simulink model "T2_Full_sim"  (R2023b)
settings: Solver=FixedStepAuto  StartTime=0.0  StopTime=Tf  FixedStep=Ts/100  MaxStep=1e-5  RelTol=1e-3
undefined symbols (not defined in the file): A_KF, AA, AAlim, Ad_KF, BB, bblim, C, C_KF, C_KF_ROT, EE, KF, KF_ROT, L, lambda_u, Mx, N, nH, plecs, R, ref_ROT, Ts, Vdc, Vo, W, w, x_ROT
libraries: spsAlphaBetaZerotoabcLib x6
settings Model: Creator=lokit  LastModifiedBy=pablo

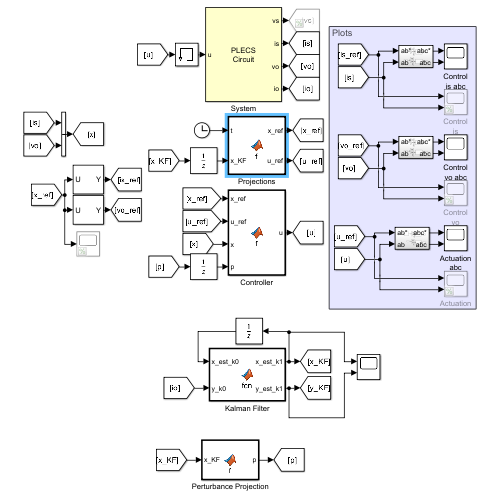
[thumbnail: Simulink's stored preview of the top-level diagram]
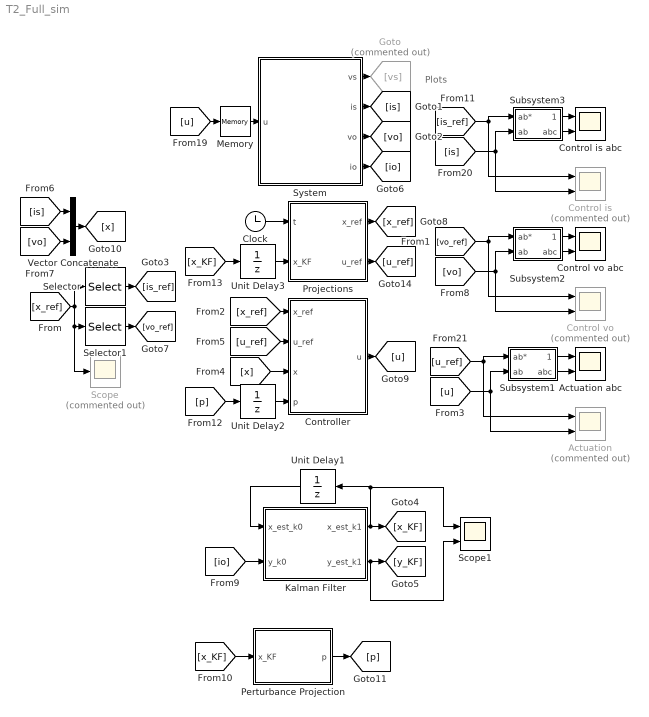
== system T2_Full_sim ==
  note: Plots
  Actuation : Scope  Commented=on  NumInputPorts=2
  Actuation abc : Scope  NumInputPorts=2
  Clock : Clock
  Control is : Scope  Commented=on  NumInputPorts=2
  Control is abc : Scope  NumInputPorts=2
  Control vo : Scope  Commented=on  NumInputPorts=2
  Control vo abc : Scope  NumInputPorts=2
  Controller : MATLAB Function  TreatAsAtomicUnit=on  SystemSampleTime=Ts
  Goto : Goto  Commented=on  GotoTag=vs
  Kalman Filter : MATLAB Function  TreatAsAtomicUnit=on  SystemSampleTime=Ts
  Memory : Memory
  Perturbance Projection : MATLAB Function  TreatAsAtomicUnit=on  SystemSampleTime=Ts
  Projections : MATLAB Function  TreatAsAtomicUnit=on  SystemSampleTime=Ts
  Scope : Scope  Commented=on
  Scope1 : Scope  NumInputPorts=2
  Selector : Selector  InputPortWidth=4*N  IndexOptions=Index vector (dialog)  Indices=[1 2]  OutputSizes=1
  Selector1 : Selector  InputPortWidth=4*N  IndexOptions=Index vector (dialog)  Indices=[3 4]  OutputSizes=1
  Subsystem1 : Subsystem
  Subsystem2 : Subsystem
  Subsystem3 : Subsystem
  System : Subsystem  LoadFcn=plecs('sl', 200);  InitFcn=plecs('sl', 214);  StartFcn=plecs('sl', 208);  StopFcn=plecs('sl', 209);  mask(PlecsCircuit){PLECSData=<binary blob, 8800 chars, not shown>}
      mask prompts: PLECSData "PLECS Data (Do not delete or modify!)"
      mask init:
      | % PLACE CUSTOM INITIALIZATIONS ABOVE
      | % DO NOT REMOVE
      | plecs('sl', 215);
      | % DO NOT REMOVE
      settings: CopyFcn=plecs('sl', 203);  DeleteFcn=plecs('sl', 205);  UndoDeleteFcn=plecs('sl', 206);  PreSaveFcn=plecs('sl', 211);  PostSaveFcn=plecs('sl', 201);  NameChangeFcn=plecs('sl', 210);  DestroyFcn=plecs('sl', 207);  PreCopyFcn=plecs('sl', 216);  OpenFcn=plecs('sl', 202);  ErrorFcn=plerrorfcn
      mask Help: eval('plecs(''help'', ''qthelp:///creatingacircuit.html'')')
      mask Display: disp('PLECS\nCircuit')
  Unit Delay1 : UnitDelay  InitialCondition=zeros(nH, 1)  SampleTime=Ts  HasFrameUpgradeWarning=on
  Unit Delay2 : UnitDelay  SampleTime=Ts  HasFrameUpgradeWarning=on
  Unit Delay3 : UnitDelay  SampleTime=Ts  HasFrameUpgradeWarning=on
  Vector Concatenate : Concatenate
  wires:
  Projections/1(x_ref) -> [x_ref]
  Clock/1 -> Projections/1(t)
  Controller/1(u) -> [u]
  [x_ref] -> Controller/1(x_ref)
  [x] -> Controller/3(x)
  [is] -> Vector Concatenate/1
  [vo] -> Vector Concatenate/2
  Vector Concatenate/1 -> [x]
  Projections/2(u_ref) -> [u_ref]
  [u_ref] -> Controller/2(u_ref)
  [u_ref] -> Subsystem1/1(ab*), Actuation/1
  Subsystem1/2(abc) -> Actuation abc/2
  Subsystem1/1(abc*) -> Actuation abc/1
  [u] -> Actuation/2, Subsystem1/2(ab)
  Selector/1 -> [is_ref]
  [x_ref] -> Scope/1, Selector1/1, Selector/1
  Subsystem2/2(abc) -> Control vo abc/2
  [vo_ref] -> Control vo/1, Subsystem2/1(ab*)
  [vo] -> Control vo/2, Subsystem2/2(ab)
  Subsystem2/1(abc*) -> Control vo abc/1
  Subsystem3/2(abc) -> Control is abc/2
  [is_ref] -> Control is/1, Subsystem3/1(ab*)
  [is] -> Subsystem3/2(ab), Control is/2
  Subsystem3/1(abc*) -> Control is abc/1
  Selector1/1 -> [vo_ref]
  System/4(io) -> [io]
  System/1(vs) -> Goto/1
  Memory/1 -> System/1(u)
  [u] -> Memory/1
  System/3(vo) -> [vo]
  System/2(is) -> [is]
  Kalman Filter/1(x_est_k1) -> Scope1/1, Unit Delay1/1, [x_KF]
  Kalman Filter/2(y_est_k1) -> Scope1/2, [y_KF]
  [io] -> Kalman Filter/2(y_k0)
  Unit Delay1/1 -> Kalman Filter/1(x_est_k0)
  [x_KF] -> Perturbance Projection/1(x_KF)
  [p] -> Unit Delay2/1
  Perturbance Projection/1(p) -> [p]
  [x_KF] -> Unit Delay3/1
  Unit Delay3/1 -> Projections/2(x_KF)
  Unit Delay2/1 -> Controller/4(p)

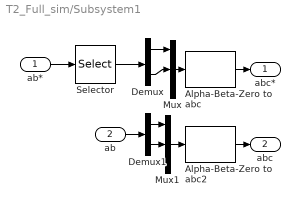
== system T2_Full_sim/Subsystem1 ==
  ab* : Inport
  ab : Inport  Port=2
  Alpha-Beta-Zero to abc : spsAlphaBetaZerotoabcLib/Alpha-Beta-Zero to abc
      settings: LibrarySourceBlock=|
      | sps_lib/Control/Alpha-Beta-Zero
      | to abc
  Alpha-Beta-Zero to abc2 : spsAlphaBetaZerotoabcLib/Alpha-Beta-Zero to abc
      settings: LibrarySourceBlock=|
      | sps_lib/Control/Alpha-Beta-Zero
      | to abc
  Demux : Demux  Outputs=2
  Demux1 : Demux  Outputs=2
  Mux : Mux  Inputs=3
  Mux1 : Mux  Inputs=3
  Selector : Selector  InputPortWidth=2*N  IndexOptions=Index vector (dialog)  Indices=[1 2]  OutputSizes=1
  abc* : Outport
  abc : Outport  Port=2
  wires:
  Demux/1 -> Mux/1
  Demux/2 -> Mux/2
  Mux/1 -> Alpha-Beta-Zero to abc/1
  ab*/1 -> Selector/1
  Mux1/1 -> Alpha-Beta-Zero to abc2/1
  Alpha-Beta-Zero to abc/1 -> abc*/1
  Alpha-Beta-Zero to abc2/1 -> abc/1
  Demux1/1 -> Mux1/1
  ab/1 -> Demux1/1
  Demux1/2 -> Mux1/2
  Selector/1 -> Demux/1

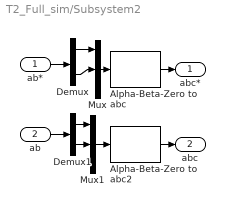
== system T2_Full_sim/Subsystem2 ==
  ab* : Inport
  ab : Inport  Port=2
  Alpha-Beta-Zero to abc : spsAlphaBetaZerotoabcLib/Alpha-Beta-Zero to abc
      settings: LibrarySourceBlock=|
      | sps_lib/Control/Alpha-Beta-Zero
      | to abc
  Alpha-Beta-Zero to abc2 : spsAlphaBetaZerotoabcLib/Alpha-Beta-Zero to abc
      settings: LibrarySourceBlock=|
      | sps_lib/Control/Alpha-Beta-Zero
      | to abc
  Demux : Demux  Outputs=2
  Demux1 : Demux  Outputs=2
  Mux : Mux  Inputs=3
  Mux1 : Mux  Inputs=3
  abc* : Outport
  abc : Outport  Port=2
  wires:
  Demux/1 -> Mux/1
  Demux/2 -> Mux/2
  Mux/1 -> Alpha-Beta-Zero to abc/1
  ab*/1 -> Demux/1
  Mux1/1 -> Alpha-Beta-Zero to abc2/1
  Alpha-Beta-Zero to abc/1 -> abc*/1
  Alpha-Beta-Zero to abc2/1 -> abc/1
  Demux1/1 -> Mux1/1
  ab/1 -> Demux1/1
  Demux1/2 -> Mux1/2

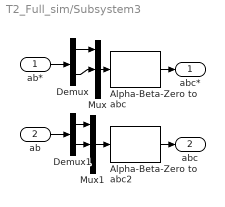
== system T2_Full_sim/Subsystem3 ==
  ab* : Inport
  ab : Inport  Port=2
  Alpha-Beta-Zero to abc : spsAlphaBetaZerotoabcLib/Alpha-Beta-Zero to abc
      settings: LibrarySourceBlock=|
      | sps_lib/Control/Alpha-Beta-Zero
      | to abc
  Alpha-Beta-Zero to abc2 : spsAlphaBetaZerotoabcLib/Alpha-Beta-Zero to abc
      settings: LibrarySourceBlock=|
      | sps_lib/Control/Alpha-Beta-Zero
      | to abc
  Demux : Demux  Outputs=2
  Demux1 : Demux  Outputs=2
  Mux : Mux  Inputs=3
  Mux1 : Mux  Inputs=3
  abc* : Outport
  abc : Outport  Port=2
  wires:
  Demux/1 -> Mux/1
  Demux/2 -> Mux/2
  Mux/1 -> Alpha-Beta-Zero to abc/1
  ab*/1 -> Demux/1
  Mux1/1 -> Alpha-Beta-Zero to abc2/1
  Alpha-Beta-Zero to abc/1 -> abc*/1
  Alpha-Beta-Zero to abc2/1 -> abc/1
  Demux1/1 -> Mux1/1
  ab/1 -> Demux1/1
  Demux1/2 -> Mux1/2

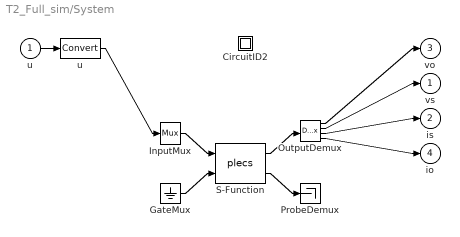
== system T2_Full_sim/System ==
  u : Inport  PortDimensions=2
  " CircuitID2 " : Subsystem
  " GateMux " : Ground
  " InputMux " : Mux  Inputs=[ 2 ]
  " OutputDemux " : Demux  Outputs=[ 2 2 2 2 ]
  " ProbeDemux " : Terminator
  " S-Function " : S-Function  FunctionName=plecs  SFunctionDeploymentMode=off  EnableBusSupport=off
  " u " : DataTypeConversion
  vs : Outport  PortDimensions=2
  is : Outport  Port=2  PortDimensions=2
  vo : Outport  Port=3  PortDimensions=2
  io : Outport  Port=4  PortDimensions=2
  wires:
  " InputMux "/1 -> " S-Function "/1
  " GateMux "/1 -> " S-Function "/2
  " S-Function "/1 -> " OutputDemux "/1
  " S-Function "/2 -> " ProbeDemux "/1
  u/1 -> " u "/1
  " u "/1 -> " InputMux "/1
  " OutputDemux "/1 -> vo/1
  " OutputDemux "/2 -> vs/1
  " OutputDemux "/3 -> is/1
  " OutputDemux "/4 -> io/1

== system T2_Full_sim/System/ CircuitID2  ==

== matlab function T2_Full_sim/Perturbance Projection ==
  data: x_KF input; KF_ROT parameter; C_KF_ROT parameter; p output
function p = f(x_KF, KF_ROT, C_KF_ROT)

p = C_KF_ROT * KF_ROT * x_KF;

== matlab function T2_Full_sim/Kalman Filter ==
  data: x_est_k0 input; x_est_k1 output; y_k0 input; Ad_KF parameter; C_KF parameter; KF parameter; y_est_k1 output
function [x_est_k1, y_est_k1] = fcn(x_est_k0, y_k0, Ad_KF, C_KF, KF)

% Entradas:
% x_est_k0: x estimada del paso inicial
% y_k0: y medida del paso inicial
% Variables
% y_est_k0: y estimada del paso inicial
% Salidas
% x_est_k1: x estimada del paso siguiente
% y_est_k1: y estimada del paso siguiente

y_est_k0 = C_KF * x_est_k0;
x_est_k1 = Ad_KF * x_est_k0 + KF * (y_k0 - y_est_k0);
y_est_k1 = C_KF * x_est_k1;

== matlab function T2_Full_sim/Projections ==
  data: t input; x_KF input; Vo parameter; w parameter; C parameter; L parameter; R parameter; x_ref output; Vdc parameter; ref_ROT parameter; Ts parameter; u_ref output; x_ROT parameter; A_KF parameter; C_KF_ROT parameter; KF_ROT parameter; C_KF parameter
function [x_ref, u_ref] = f(t, x_KF, Vo, w, C, L, R, Vdc, ref_ROT, Ts, x_ROT, A_KF, C_KF_ROT, KF_ROT, C_KF)
theta = w * t;
theta_1 = theta + w * Ts;
%% u_ref (instantly)
% vs = io(R+pL) + vo*(1+pRC+p^2*LC)
% vs = vs_io + vs_vo
vs_vo = 2/3 * Vo * ((1-w^2*L*C)*[cos(theta); sin(theta)] + w*R*C*[-sin(theta); cos(theta)]); % vs_vo[k]
vs_vo = ref_ROT * vs_vo; % vs_vo[k:k+N-1]
vs_io = C_KF_ROT * KF_ROT * (R + L * A_KF) * x_KF; % vs_io[k:k+N-1]
vs_ref = vs_io + vs_vo;
u_ref = vs_ref * 3 / Vdc;
%% x_ref
vo_ref = Vo * [cos(theta_1); sin(theta_1)]; % vo[k+1]
% is = io + C * (d/dt) * vo
% is = is_io + is_vo
pvo_ref = w * Vo * [-sin(theta_1); cos(theta_1)]; % pvo[k+1]
is_ref= C_KF * x_KF + C *  pvo_ref; % is[k+1]
x_ref_aux = [is_ref; vo_ref]; % x[k]
x_ref = x_ROT * x_ref_aux; %????

== matlab function T2_Full_sim/Controller ==
  data: x_ref input; u_ref input; x input; p input; u output; W parameter; AAlim parameter; bblim parameter; AA parameter; lambda_u parameter; BB parameter; Mx parameter; EE parameter
function u = f(x_ref, u_ref, x, p, W, AAlim, bblim, AA, lambda_u, BB, Mx, EE)

coder.extrinsic('quadprog')

x0 = x;

Fx = (BB.') * (Mx.') * (-x_ref + AA * x0 + EE * p);
Fu = -2 * u_ref;
F = Fx + lambda_u * Fu;

U = quadprog(W, F, AAlim, bblim);

u = zeros(2, 1);
u = U(1:2);
